simulink subsystem "OrbitalDynamics"  (R2023a)
settings: Solver=VariableStepAuto  StartTime=0.0  StopTime=10.0  RelTol=1e-3
undefined symbols (not defined in the file or in its folder): Earth
settings Model: Creator=Andy  LastModifiedBy=Andy

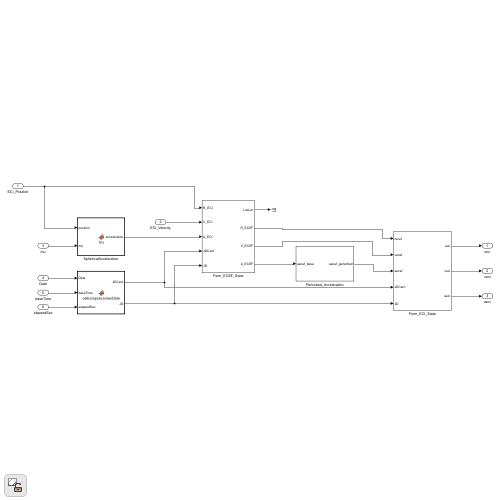
[thumbnail: Simulink's stored preview of the top-level diagram]
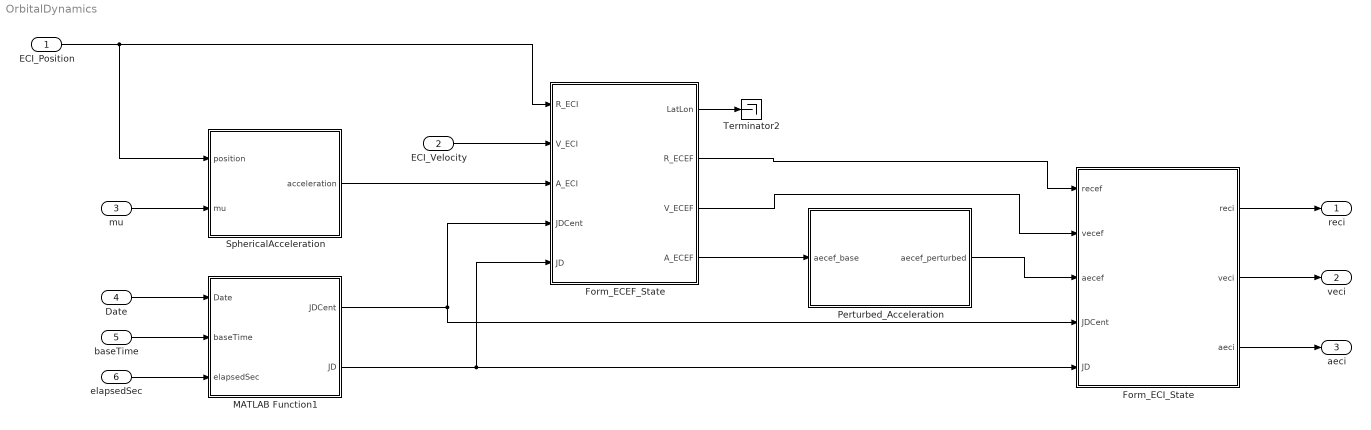
== system OrbitalDynamics ==
  ECI_Position : Inport
  ECI_Velocity : Inport  Port=2
  mu : Inport  Port=3
  Date : Inport  Port=4
  baseTime : Inport  Port=5
  elapsedSec : Inport  Port=6
  Form_ECEF_State : Subsystem
  Form_ECI_State : Subsystem
  MATLAB Function1 : MATLAB Function  TreatAsAtomicUnit=on
  Perturbed_Acceleration : Subsystem
  SphericalAcceleration : MATLAB Function  TreatAsAtomicUnit=on
  Terminator2 : Terminator
  reci : Outport
  veci : Outport  Port=2
  aeci : Outport  Port=3
  wires:
  Form_ECEF_State/2(R_ECEF) -> Form_ECI_State/1(recef)
  MATLAB Function1/1(JDCent) -> Form_ECI_State/4(JDCent), Form_ECEF_State/4(JDCent)
  SphericalAcceleration/1(acceleration) -> Form_ECEF_State/3(A_ECI)
  ECI_Position/1 -> SphericalAcceleration/1(position), Form_ECEF_State/1(R_ECI)
  Form_ECEF_State/1(LatLon) -> Terminator2/1
  elapsedSec/1 -> MATLAB Function1/3(elapsedSec)
  Perturbed_Acceleration/1(aecef_perturbed) -> Form_ECI_State/3(aecef)
  Date/1 -> MATLAB Function1/1(Date)
  MATLAB Function1/2(JD) -> Form_ECI_State/5(JD), Form_ECEF_State/5(JD)
  Form_ECEF_State/3(V_ECEF) -> Form_ECI_State/2(vecef)
  Form_ECEF_State/4(A_ECEF) -> Perturbed_Acceleration/1(aecef_base)
  Form_ECI_State/1(reci) -> reci/1
  ECI_Velocity/1 -> Form_ECEF_State/2(V_ECI)
  Form_ECI_State/3(aeci) -> aeci/1
  mu/1 -> SphericalAcceleration/2(mu)
  Form_ECI_State/2(veci) -> veci/1
  baseTime/1 -> MATLAB Function1/2(baseTime)

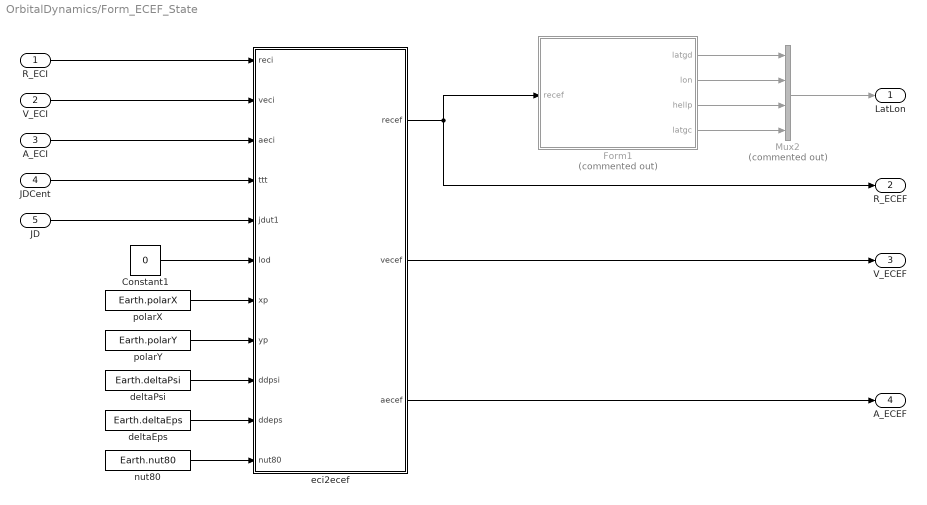
== system OrbitalDynamics/Form_ECEF_State ==
  R_ECI : Inport  OutDataTypeStr=double  PortDimensions=3
  V_ECI : Inport  Port=2  OutDataTypeStr=double  PortDimensions=3
  A_ECI : Inport  Port=3  OutDataTypeStr=double  PortDimensions=3
  JDCent : Inport  Port=4  OutDataTypeStr=double
  JD : Inport  Port=5  OutDataTypeStr=double
  Constant1 : Constant  Value=0
  Form1 : MATLAB Function  Commented=on  TreatAsAtomicUnit=on
  Mux2 : Mux  Commented=on
  deltaEps : Constant  Value=Earth.deltaEps
  deltaPsi : Constant  Value=Earth.deltaPsi
  eci2ecef : MATLAB Function  TreatAsAtomicUnit=on
  nut80 : Constant  Value=Earth.nut80
  polarX : Constant  Value=Earth.polarX
  polarY : Constant  Value=Earth.polarY
  LatLon : Outport
  R_ECEF : Outport  Port=2
  V_ECEF : Outport  Port=3
  A_ECEF : Outport  Port=4
  wires:
  eci2ecef/3(aecef) -> A_ECEF/1
  A_ECI/1 -> eci2ecef/3(aeci)
  JD/1 -> eci2ecef/5(jdut1)
  JDCent/1 -> eci2ecef/4(ttt)
  nut80/1 -> eci2ecef/11(nut80)
  Form1/4(latgc) -> Mux2/4
  deltaPsi/1 -> eci2ecef/9(ddpsi)
  eci2ecef/1(recef) -> Form1/1(recef), R_ECEF/1
  R_ECI/1 -> eci2ecef/1(reci)
  Form1/2(lon) -> Mux2/2
  deltaEps/1 -> eci2ecef/10(ddeps)
  polarX/1 -> eci2ecef/7(xp)
  V_ECI/1 -> eci2ecef/2(veci)
  Mux2/1 -> LatLon/1
  Form1/1(latgd) -> Mux2/1
  polarY/1 -> eci2ecef/8(yp)
  Constant1/1 -> eci2ecef/6(lod)
  Form1/3(hellp) -> Mux2/3
  eci2ecef/2(vecef) -> V_ECEF/1

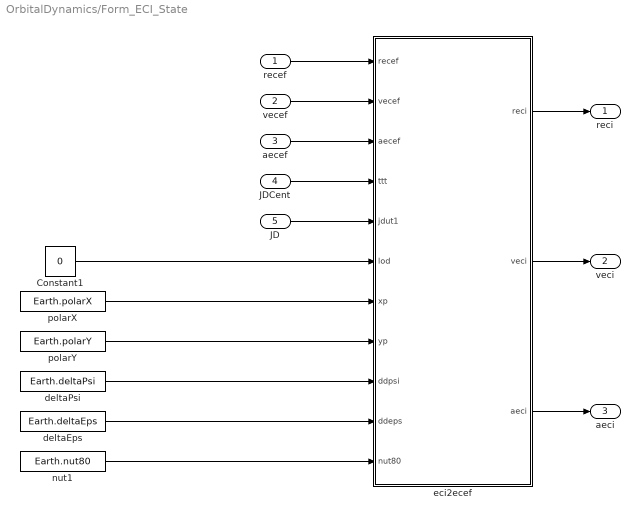
== system OrbitalDynamics/Form_ECI_State ==
  recef : Inport
  vecef : Inport  Port=2
  aecef : Inport  Port=3
  JDCent : Inport  Port=4  OutDataTypeStr=double
  JD : Inport  Port=5  OutDataTypeStr=double
  Constant1 : Constant  Value=0
  deltaEps : Constant  Value=Earth.deltaEps
  deltaPsi : Constant  Value=Earth.deltaPsi
  eci2ecef : MATLAB Function  TreatAsAtomicUnit=on
  nut1 : Constant  Value=Earth.nut80
  polarX : Constant  Value=Earth.polarX
  polarY : Constant  Value=Earth.polarY
  reci : Outport
  veci : Outport  Port=2
  aeci : Outport  Port=3
  wires:
  JD/1 -> eci2ecef/5(jdut1)
  JDCent/1 -> eci2ecef/4(ttt)
  eci2ecef/3(aeci) -> aeci/1
  aecef/1 -> eci2ecef/3(aecef)
  deltaPsi/1 -> eci2ecef/9(ddpsi)
  recef/1 -> eci2ecef/1(recef)
  vecef/1 -> eci2ecef/2(vecef)
  Constant1/1 -> eci2ecef/6(lod)
  deltaEps/1 -> eci2ecef/10(ddeps)
  eci2ecef/1(reci) -> reci/1
  polarX/1 -> eci2ecef/7(xp)
  eci2ecef/2(veci) -> veci/1
  nut1/1 -> eci2ecef/11(nut80)
  polarY/1 -> eci2ecef/8(yp)

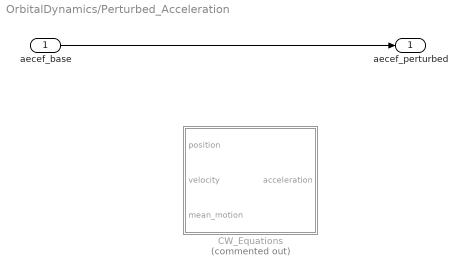
== system OrbitalDynamics/Perturbed_Acceleration ==
  aecef_base : Inport
  CW_Equations : MATLAB Function  Commented=on  TreatAsAtomicUnit=on
  aecef_perturbed : Outport
  wires:
  aecef_base/1 -> aecef_perturbed/1

== matlab function OrbitalDynamics/Form_ECEF_State/Form1 ==
  data: recef input; latgd output; lon output; hellp output; latgc output
function [latgd,lon,hellp,latgc] = callijk2ll(recef)


[latgc,latgd,lon,hellp] = ijk2ll ( recef );

== matlab function OrbitalDynamics/Form_ECEF_State/eci2ecef ==
  data: reci input; recef output; veci input; aeci input; ttt input; jdut1 input; lod input; xp input; yp input; ddpsi input; ddeps input; vecef output; nut80 input; aecef output
function [recef, vecef, aecef] = calleci2ecef(reci,veci,aeci,ttt,jdut1,lod,xp,yp,ddpsi,ddeps,nut80)

% Use additional sidereal time terms
eqeterms = 1;

% Function expects km, i/o is in m
[recef,vecef,aecef] = eci2ecef(reci/1000,veci/1000,aeci/1000,ttt,jdut1,lod,xp,yp,eqeterms,ddpsi,ddeps,nut80 );
recef = recef*1000;
vecef = vecef*1000;
aecef = aecef*1000;

== matlab function OrbitalDynamics/Form_ECI_State/eci2ecef ==
  data: recef input; reci output; vecef input; aecef input; ttt input; jdut1 input; lod input; xp input; yp input; ddpsi input; ddeps input; veci output; nut80 input; aeci output
function [reci, veci, aeci] = callecef2eci(recef,vecef,aecef,ttt,jdut1,lod,xp,yp,ddpsi,ddeps,nut80)


% Use additional sidereal time terms
eqeterms = 1;

% Function expects km, i/o is in m
[reci,veci,aeci] = ecef2eci( recef/1000,vecef/1000,aecef/1000,ttt,jdut1,lod,xp,yp,eqeterms,ddpsi,ddeps,nut80 );
reci = reci*1000;
veci = veci*1000;
aeci = aeci*1000;

== matlab function OrbitalDynamics/MATLAB Function1 ==
  data: JDCent output; Date input; JD output; baseTime input; elapsedSec input
function [JDCent, JD] = callcomputeJulianDate(Date,baseTime,elapsedSec)

% Form the current time vector
Time = baseTime + [0 0 elapsedSec]';

% Get the Julian Date
JD = computeJulianDate(Date,Time);

% Compute the elapsed Julian Centuries from epoch (J2000)
JDCent = (JD - 2451545.0) / 36525;

== matlab function OrbitalDynamics/Perturbed_Acceleration/CW_Equations ==
  data: position input; acceleration output; velocity input; mean_motion input
function acceleration = fcn(position,velocity,mean_motion)

acceleration = [( 2*mean_motion*velocity(2) + 3*mean_motion^2*position(1)) ...
                 -2*mean_motion*velocity(1) ...
                 -1*mean_motion^2*position(3)];

== matlab function OrbitalDynamics/SphericalAcceleration ==
  data: position input; acceleration output; mu input
function acceleration = fcn(position,mu)

rmag = norm(position);
acceleration = -mu/rmag^2 * position/rmag;
